simulink model "HV_TableLookup_T5"  (R2025a)
settings: Solver=ode23tb  StartTime=0.0  StopTime=1000  MaxStep=0.1  RelTol=1e-3
settings Model: DataDictionary=FuelGaugingData.sldd  Creator=mkelley  LastModifiedBy=mkelley

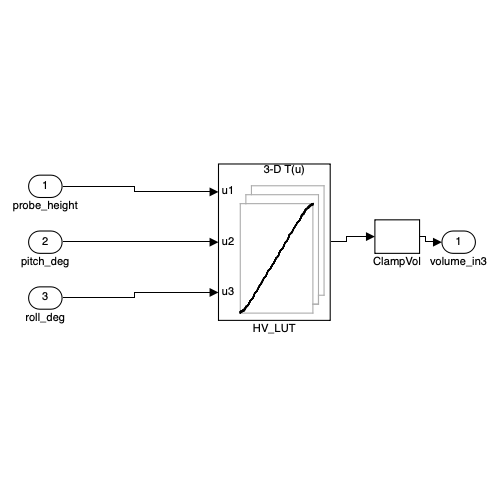
[thumbnail: Simulink's stored preview of the top-level diagram]
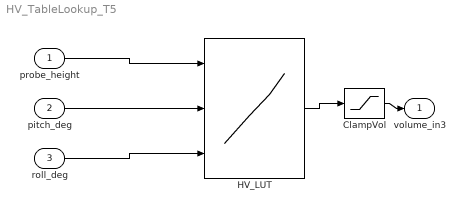
== system HV_TableLookup_T5 ==
  probe_height : Inport
  pitch_deg : Inport  Port=2
  roll_deg : Inport  Port=3
  ClampVol : Saturate  UpperLimit=inf  LowerLimit=0
  HV_LUT : Lookup_n-D  NumberOfTableDimensions=3  DataSpecification=Lookup table object  LookupTableObject=LUT_T5  BreakpointsForDimension3=[5, 7]  Table=reshape(repmat([4 5 6;16 19 20;10 18 23],1,2),[3,3,2])  ExtrapMethod=Clip  InternalRulePriority=Speed  RndMeth=Simplest
      settings: InputPortMap=u0,u1,u2
  volume_in3 : Outport
  wires:
  probe_height/1 -> HV_LUT/1
  pitch_deg/1 -> HV_LUT/2
  roll_deg/1 -> HV_LUT/3
  HV_LUT/1 -> ClampVol/1
  ClampVol/1 -> volume_in3/1
